simulink model "pmsg_wind_turbine_PI"  (R2022a)
settings: Solver=ode23tb  StartTime=0.0  StopTime=30  FixedStep=1e-4  MaxStep=1e-6  RelTol=1e-3
values from neighbouring files (symbols this model uses):
  Ci = 2878*10^-6    (= 0.002878)    [Completo.m]
  Lb = 0.9513*10^-3    (= 0.0009513)    [Completo.m]
  time = dados.Time;n    [Completo.m]
  vwind = dados.Vvento    [Completo.m]
undefined symbols (not defined in the file or in its folder): sigbuilder_block
libraries: spsCurrentMeasurementLib x3, eePowerMeasurement x3, spsVoltageMeasurementLib x3, spsSeriesRLCBranchLib x2, spsDCVoltageSourceLib x1, spsDiodeLib x1, spsMosfetLib x1, slpidlib x1, spsPWMGeneratorDCDCLib x1, spsPermanentMagnetSynchronousMachineLib x1, spsThreePhaseVIMeasurementLib x1, spsUniversalBridgeLib x1
settings Model: Creator=Taysa Banik  LastModifiedBy=LICON
settings SolverCC: ZeroCrossAlgorithm=Adaptive
settings DebuggingCC: MaxConsecutiveZCsMsg=warning  MaskedZcDiagnostic=none  IgnoredZcDiagnostic=none  MultiTaskCondExecSysMsg=warning  MultiTaskRateTransMsg=warning  ModelReferenceExtraNoncontSigs=warning

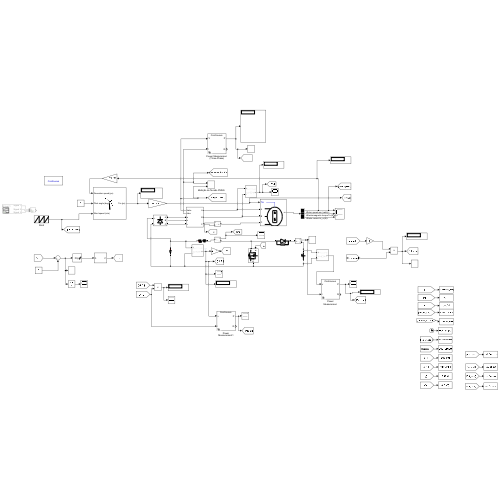
[thumbnail: Simulink's stored preview of the top-level diagram]
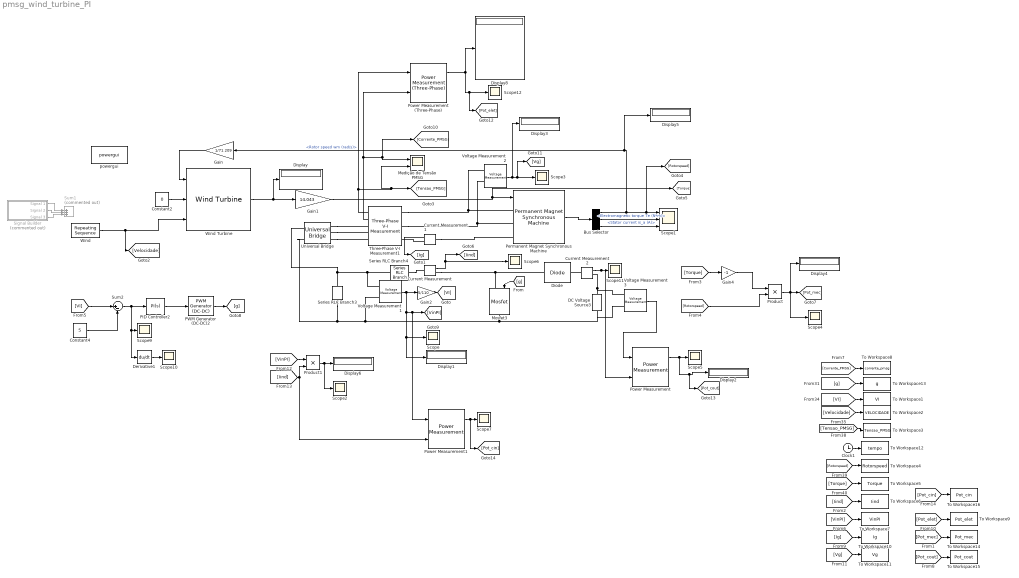
== system pmsg_wind_turbine_PI ==
  Bus Selector : BusSelector  OutputSignals=Rotor speed wm (rad/s),Electromagnetic torque Te (N*m),Stator current is_a (A)
  Clock1 : Clock
  Constant2 : Constant  Value=0
  Constant4 : Constant  Value=5
  Current Measurement : spsCurrentMeasurementLib/Current Measurement  PhasorSimulation=off  OutputType=Complex  PSBequivalent=0
  Current Measurement1 : spsCurrentMeasurementLib/Current Measurement  PhasorSimulation=off  OutputType=Complex  PSBequivalent=0
  Current Measurement2 : spsCurrentMeasurementLib/Current Measurement  PhasorSimulation=off  OutputType=Complex  PSBequivalent=0
  DC Voltage Source3 : spsDCVoltageSourceLib/DC Voltage Source  Amplitude=400  Measurements=Voltage
  Derivative1 : Derivative
  Diode : spsDiodeLib/Diode  Ron=0.001  Lon=0  Vf=0.1  IC=0  UseSnubber=0  Rs=50000  Cs=inf  Measurements=off
  Display{,1..6,8} (8 alike) : Display
  Gain : Gain  Gain=1/71.209
  Gain1 : Gain  Gain=14.043
  Gain2 : Gain  Gain=5/110
  Gain4 : Gain  Gain=-1
  Medição de Tensão PMSG : Scope  NumInputPorts=2
  Mosfet3 : spsMosfetLib/Mosfet  Ron=0.001  Lon=0  Rd=0.01  Vfd=0  IC=0  Rs=1e5  Cs=inf  Measurements=off
  PID Controller2 : slpidlib/PID Controller  Controller=PI  Form=Parallel  TimeDomain=Continuous-time  UseExternalTs=off  SampleTime=-1  IntegratorMethod=Forward Euler  FilterMethod=Forward Euler  ControllerParametersSource=internal  P=0.1928  I=11.6277  UseKiTs=off  D=0  N=100  UseFilter=on  TunerSelectOption=Frequency Response Based  InitialConditionSource=internal  InitialConditionForIntegrator=0  InitialConditionForFilter=0  DifferentiatorICPrevScaledInput=0  ExternalReset=none  TrackingMode=off  Kt=1  LimitOutput=on  SatLimitsSource=internal  UpperSaturationLimit=0.95  LowerSaturationLimit=0  LinearizeAsGain=on  AntiWindupMode=none  Kb=1  POutMin=[]  POutMax=[]  IOutMin=[]  IOutMax=[]  DOutMin=[]  DOutMax=[]  NOutMin=[]  NOutMax=[]  SumOutMin=[]  SumOutMax=[]  SaturationOutMin=[]  SaturationOutMax=[]  PParamMin=[]  PParamMax=[]  IParamMin=[]  IParamMax=[]  DParamMin=[]  DParamMax=[]  NParamMin=[]  NParamMax=[]  KbParamMin=[]  KbParamMax=[]  KtParamMin=[]  KtParamMax=[]  KbOutMin=[]  KbOutMax=[]  KtOutMin=[]  KtOutMax=[]  IntegratorOutMin=[]  IntegratorOutMax=[]  FilterOutMin=[]  FilterOutMax=[]  SumI1OutMin=[]  SumI1OutMax=[]  SumI2OutMin=[]  SumI2OutMax=[]  SumI3OutMin=[]  SumI3OutMax=[]  SumI4OutMin=[]  SumI4OutMax=[]  SumDOutMin=[]  SumDOutMax=[]  DifferentiatorOutMin=[]  DifferentiatorOutMax=[]  FilterDiffOutCoefMin=[]  FilterDiffOutCoefMax=[]  ReciprocalOutMin=[]  ReciprocalOutMax=[]  SumDenOutMin=[]  SumDenOutMax=[]  SumNumOutMin=[]  SumNumOutMax=[]  DivideOutMin=[]  DivideOutMax=[]  UdiffTsProdOutMin=[]  UdiffTsProdOutMax=[]  NTsProdOutMin=[]  NTsProdOutMax=[]  UintegralTsProdOutMin=[]  UintegralTsProdOutMax=[]  UngainTsProdOutMin=[]  UngainTsProdOutMax=[]  IntegratorContinuousStateAttributes=''  IntegratorStateMustResolveToSignalObject=off  IntegratorRTWStateStorageClass=Auto  FilterContinuousStateAttributes=''  FilterStateMustResolveToSignalObject=off  FilterRTWStateStorageClass=Auto  ParallelPVariant=InternalParameters  IdealPVariant=Disabled  IVariant=InternalParameters  DVariant=Disabled  IntegratorVariant=Continuous  SatVariant=Enabled  AWVariant=Passthrough  PCopyVariant=Disabled  TRVariant=Disabled  FdbkBlocksVariant=Forward  IdealPFdbkVariant=Disabled  SatFdbkVariant=Disabled  DerivativeFilterVariant=Disabled  NVariant=Disabled  NCopyVariant=Disabled_SignalSpec  FilterICVariant=Disabled  IntegratorICVariant=InternalICs  ExternalResetVariant=Disabled  TRSumVariant=Passthrough  SumFdbkVariant=Disabled  SumVariant=Sum_PI  TsampFilterVariant=InternalTs  TsampNgainVariant=Passthrough  TsampIntegralVariant=Passthrough  ExternalSaturationOutDataTypeStr=Inherit: Same as second input  aMode=0
  PWM Generator (DC-DC)2 : spsPWMGeneratorDCDCLib/PWM Generator (DC-DC)  Fsw=30000  Ts=1e-6
  Permanent Magnet Synchronous Machine : spsPermanentMagnetSynchronousMachineLib/Permanent Magnet Synchronous Machine  NbPhases=3  FluxDistribution=Sinusoidal  RotorType=Round  MechanicalLoad=Torque Tm  PresetModel=No  ShowDetailedParameters=on  MeasurementBus=off  Resistance=0.732  Inductance=8.5e-3  dqInductances=[8.5e-3,8.5e-3]  La=3.5e-3  MachineConstant=Voltage Constant (V_peak L-L / krpm)  Flux=0.13618  VoltageCst=172.9  TorqueCst=1.4299  Flat=120  Mechanical=[1E-3 1.79E-4 7 1E-3]  PolePairs=4  InitialConditions=[42.72,0, 0,0]  InitialConditions5ph=[0 0 0 0 0 0]  RefAngle=Aligned with phase A axis (original Park)  IterativeDiscreteModel=Trapezoidal non iterative  TsBlock=-1  TsPowergui=0
  Power Measurement : eePowerMeasurement/Power Measurement  LabelModeActiveChoice=Continuous  F=79.33  K=[0]  Ts=0
      settings: SourceProductBaseCode=PS
  Power Measurement1 : eePowerMeasurement/Power Measurement  LabelModeActiveChoice=Continuous  F=79.33  K=[0]  Ts=0
      settings: SourceProductBaseCode=PS
  Power Measurement (Three-Phase) : eePowerMeasurement/Power Measurement (Three-Phase)  LabelModeActiveChoice=Continuous  F=79.33  K=[0 1 2 3]  Seq=Positive  Ts=0
      settings: SourceProductBaseCode=PS
  Product : Product
  Product1 : Product
  Scope{,2..7,9..12} (11 alike) : Scope
  Scope1 : Scope  NumInputPorts=3
  Series RLC Branch3 : spsSeriesRLCBranchLib/Series RLC Branch  LConnTagsString=__new0  RConnTagsString=__new0  BranchType=C  Resistance=1  Inductance=1e-3  SetiL0=off  InitialCurrent=0  Capacitance=Ci  Setx0=on  InitialVoltage=100  Measurements=None
  Series RLC Branch4 : spsSeriesRLCBranchLib/Series RLC Branch  LConnTagsString=__new0  RConnTagsString=__new0  BranchType=RL  Resistance=1  Inductance=Lb  SetiL0=off  InitialCurrent=0  Capacitance=1e-3  Setx0=off  InitialVoltage=0  Measurements=None
  Signal Builder : Subsystem  Tag=STV Subsys  Commented=on  LoadFcn=sigbuilder_block('load');  StartFcn=sigbuilder_block('start');  StopFcn=sigbuilder_block('stop');  ClipboardFcn=sigbuilder_block('clipboard');  mask(Sigbuilder block){tuvar=[0:10]}
      mask help: Simulink:masks:SigbuilderBlock_MD
      mask init:
      | if ~strcmp(get_param(bdroot(gcbh),'SimulationStatus'),'stopped') tuvar = sigbuilder_block('maskInit'); end
      settings: CopyFcn=sigbuilder_block('copy');  DeleteFcn=sigbuilder_block('delete');  ModelCloseFcn=sigbuilder_block('modelClose');  PreSaveFcn=sigbuilder_block('preSave');  PauseFcn=sigbuilder_block('pause');  ContinueFcn=sigbuilder_block('continue');  NameChangeFcn=sigbuilder_block('namechange');  OpenFcn=sigbuilder_block('open',[61.5 90 1012.5 506.25 ]);  CloseFcn=sigbuilder_block('close');
      mask Display: plot(0, 0, 100, 100,[2, 2, 32, 32, 2], [68, 8, 8, 68, 68],[32, 2], [38, 38], [32, 19, 2],[53, 60, 44], [32, 17, 17, 2],[16, 16, 31, 31]);txt = getActiveGroup(gcbh);text(2, 100, txt,'verticalAlignment', 'top');
  Sum1 : Sum  Commented=on  Inputs=|+++
  Sum2 : Sum  Inputs=|+-
  Three-Phase V-I Measurement1 : spsThreePhaseVIMeasurementLib/Three-Phase V-I Measurement  VoltageMeasurement=phase-to-phase  SetLabelV=off  LabelV=Vabc  Vpu=off  VpuLL=off  CurrentMeasurement=yes  SetLabelI=off  LabelI=Iabc  Ipu=off  Pbase=100e6  Vbase=500e3  OutputType=Complex  PhasorSimulation=off  PSBequivalent=0
  To Workspace1 : ToWorkspace  VariableName=VI  SampleTime=1e-6
  To Workspace10 : ToWorkspace  VariableName=Ig  SampleTime=1e-6
  To Workspace11 : ToWorkspace  VariableName=Vg  SampleTime=1e-6
  To Workspace12 : ToWorkspace  VariableName=tempo  SampleTime=1e-6
  To Workspace13 : ToWorkspace  VariableName=g  SampleTime=1e-6
  To Workspace14 : ToWorkspace  VariableName=Pot_mec  SampleTime=1e-6
  To Workspace15 : ToWorkspace  VariableName=Pot_cout  SampleTime=1e-6
  To Workspace16 : ToWorkspace  VariableName=Pot_cin  SampleTime=1e-6
  To Workspace2 : ToWorkspace  VariableName=VELOCIDADE  SampleTime=1e-6
  To Workspace3 : ToWorkspace  VariableName=Tensao_PMSG  SampleTime=1e-6
  To Workspace4 : ToWorkspace  VariableName=Rotorspeed  SampleTime=1e-6
  To Workspace5 : ToWorkspace  VariableName=Torque  SampleTime=1e-6
  To Workspace6 : ToWorkspace  VariableName=Iind  SampleTime=1e-6
  To Workspace7 : ToWorkspace  VariableName=VinPI  SampleTime=1e-6
  To Workspace8 : ToWorkspace  VariableName=corrente_pmsg  SampleTime=1e-6
  To Workspace9 : ToWorkspace  VariableName=Pot_elet  SampleTime=1e-6
  Universal Bridge : spsUniversalBridgeLib/Universal Bridge  Arms=3  SnubberResistance=100000  SnubberCapacitance=inf  Device=Diodes  Ron=1e-3  Lon=0  ForwardVoltages="[  0  0  ]"  ForwardVoltage=0.1  GTOparameters=[ 10e-6 , 20e-6 ]  IGBTparameters=[ 1e-6 , 2e-6 ]  Measurements=None  Measurements_2=None  converterType=Rectifier
  Voltage Measurement1 : spsVoltageMeasurementLib/Voltage Measurement  PhasorSimulation=off  OutputType=Complex  PSBequivalent=0
  Voltage Measurement2 : spsVoltageMeasurementLib/Voltage Measurement  PhasorSimulation=off  OutputType=Complex  PSBequivalent=0
  Voltage Measurement3 : spsVoltageMeasurementLib/Voltage Measurement  PhasorSimulation=off  OutputType=Complex  PSBequivalent=0
  Wind : simulink/Sources/Repeating Sequence  rep_seq_t=[time]  rep_seq_y=[vwind]
  Wind Turbine : spsWindTurbineLib/Wind Turbine  Pnom=1000  Pelec_base=1000  wind_base=12  P_wind_base=1  speed_nom=1  pitch_angle=0  c1_c6="[0.51763          116          0.4            5           21     0.006795]"  cp_nom=0.48  lambda_nom=8.1
      settings: SourceProductBaseCode=PS
  powergui : spspowerguiLib/powergui  Priority=1  SimulationMode=Continuous  SampleTime=50e-6  frequency=60  Iterations=50  frequencyindice=0  Pbase=100e6  ErrMax=1e-4  UnitsV=kV  UnitsW=MW  buscounter=0  FunctionMessages=off  echomessages=off  EnableUseOfTLC=off  CurrentSourceSwitches=off  DisableSnubberDevices=off  DisableRonSwitches=off  DisableVfSwitches=off  DisplayEquations=off  AutomaticDiscreteSolvers=off  SolverType=Tustin/Backward Euler (TBE)  Interpol=off  ExternalGateDelay=off  methode=off  Ts=100  x0status=blocks  SPID=on  SwTol=0  HookPort=off  NonlinearTolerance=1e-4  nMaxIteration=100  ContinueOnMaxIteration=off  RestoreLinks=warning  ResistiveCurrentMeasurement=off  Frange=[0:2:500]  Ylog=off  Xlog=on  ShowGrid=off  save=off  variable=ZData  structure=0  ZoomFFT=off  StartTime=0.0  cycles=1  DisplayStyle=1  fundamental=60  FreqAxis=off  MaxFrequency=1000  frequencyindicesteady=1  RmsSteady=1  display=off
  wires:
  Constant2/1 -> Wind Turbine/2
  Three-Phase V-I Measurement1/1 -> Power Measurement (Three-Phase)/1, Medição de Tensão PMSG/2, [Tensao_PMSG]
  Permanent Magnet Synchronous Machine/1 -> Bus Selector/1
  Bus Selector/1 -> [Rotorspeed], Scope1/1, Display5/1, Gain/1  "<Rotor speed wm (rad/s)>"
  Bus Selector/2 -> Scope1/2  "<Electromagnetic torque Te (N*m)>"
  Bus Selector/3 -> Scope1/3  "<Stator current is_a (A)>"
  Gain/1 -> Wind Turbine/1
  Wind Turbine/1 -> Display/1, Gain1/1
  Gain1/1 -> Permanent Magnet Synchronous Machine/1, [Torque]
  Voltage Measurement1/1 -> Gain2/1, Power Measurement1/1, [VinPI], Scope/1, Display1/1
  [g] -> Mosfet3/1
  Gain2/1 -> [VI]
  Signal Builder/1(Signal 1) -> Sum1/1
  Signal Builder/2(Signal 2) -> Sum1/2
  Signal Builder/3(Signal 3) -> Sum1/3
  [VI] -> To Workspace1/1
  [g] -> To Workspace13/1
  [Torque] -> To Workspace5/1
  [Velocidade] -> To Workspace2/1
  Clock1/1 -> To Workspace12/1
  [Tensao_PMSG] -> To Workspace3/1
  [Rotorspeed] -> To Workspace4/1
  Current Measurement/1 -> [Iind], Scope6/1
  [Iind] -> To Workspace6/1
  Product/1 -> Display4/1, Scope4/1, [Pot_mec]
  [Rotorspeed] -> Product/2
  [Torque] -> Gain4/1
  Gain4/1 -> Product/1
  Constant4/1 -> Sum2/2
  [VI] -> Sum2/1
  PID Controller2/1 -> PWM Generator (DC-DC)2/1
  Derivative1/1 -> Scope10/1
  PWM Generator (DC-DC)2/1 -> [g]
  Sum2/1 -> Derivative1/1, Scope9/1, PID Controller2/1
  [VinPI] -> To Workspace7/1
  [Corrente_PMSG] -> To Workspace8/1
  [Pot_elet] -> To Workspace9/1
  Current Measurement1/1 -> [Ig]
  Voltage Measurement2/1 -> Display3/1, [Vg], Scope3/1
  [Vg] -> To Workspace11/1
  [Ig] -> To Workspace10/1
  [Pot_mec] -> To Workspace14/1
  Current Measurement2/1 -> Power Measurement/2, Scope11/1
  Power Measurement (Three-Phase)/1 -> [Pot_elet], Scope12/1, Display8/1
  Three-Phase V-I Measurement1/2 -> Power Measurement (Three-Phase)/2, Medição de Tensão PMSG/1, [Corrente_PMSG]
  Voltage Measurement3/1 -> Power Measurement/1
  Power Measurement/1 -> [Pot_cout], Display2/1, Scope5/1
  [Pot_cout] -> To Workspace15/1
  [Iind] -> Product1/2, Power Measurement1/2
  Product1/1 -> Scope2/1, Display6/1
  Wind/1 -> [Velocidade], Wind Turbine/3
  [VinPI] -> Product1/1
  Power Measurement1/1 -> [Pot_cin], Scope7/1
  [Pot_cin] -> To Workspace16/1
  connections:
  Three-Phase V-I Measurement1/LConn1 -- Voltage Measurement2/LConn1 -- Permanent Magnet Synchronous Machine/LConn1
  Three-Phase V-I Measurement1/LConn2 -- Voltage Measurement2/LConn2 -- Permanent Magnet Synchronous Machine/LConn2
  Universal Bridge/LConn1 -- Three-Phase V-I Measurement1/RConn1
  Universal Bridge/LConn2 -- Three-Phase V-I Measurement1/RConn2
  Universal Bridge/LConn3 -- Three-Phase V-I Measurement1/RConn3
  Mosfet3/LConn1 -- Current Measurement/RConn1 -- Diode/LConn1
  Voltage Measurement1/LConn1 -- Series RLC Branch4/LConn1 -- Universal Bridge/RConn1 -- Series RLC Branch3/LConn1
  Series RLC Branch3/RConn1 -- Universal Bridge/RConn2 -- Voltage Measurement1/LConn2 -- Voltage Measurement3/LConn2 -- DC Voltage Source3/LConn1 -- Mosfet3/RConn1
  Current Measurement1/LConn1 -- Permanent Magnet Synchronous Machine/LConn3
  Current Measurement1/RConn1 -- Three-Phase V-I Measurement1/LConn3
  Series RLC Branch4/RConn1 -- Current Measurement/LConn1
  Current Measurement2/LConn1 -- Diode/RConn1
  DC Voltage Source3/RConn1 -- Current Measurement2/RConn1 -- Voltage Measurement3/LConn1

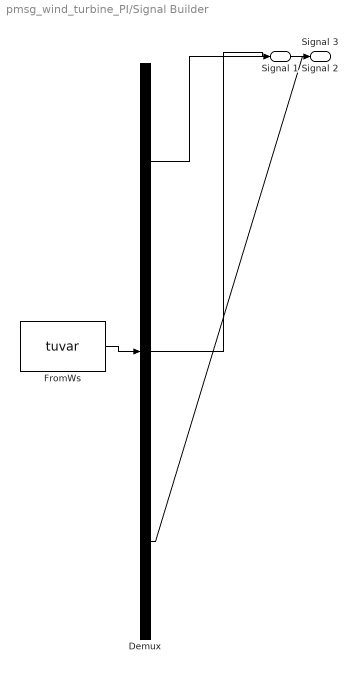
== system pmsg_wind_turbine_PI/Signal Builder ==
  Demux : Demux  Tag=STV Demux  Outputs=3
      settings: DisplayOption=none
  FromWs : FromWorkspace  Tag=STV FromWs  VariableName=tuvar
      SigBuilderData=|
      | common.afterFinalStr = 'Extrapolate'
      | common.sampleTime = 0
      | dataSet.timeRange = [0 10]
      | dataSet.name = 'Group 1'
      | sbobj.Groups.Name = 'Group 1'
      | sbobj.Groups.Signals(1).Name = 'Signal 1'
      | sbobj.Groups.Signals(1).XData = [0 1.5 1.5 6 10]
      | sbobj.Groups.Signals(1).YData = [12 12 0 0 0]
      | sbobj.Groups.Signals(2).Name = 'Signal 2'
      | sbobj.Groups.Signals(2).XData = [0 1.5 1.5 2.5 2.5 10]
      | sbobj.Groups.Signals(2).YData = [0 0 10 10 0 0]
      | sbobj.Groups.Signals(3).Name = 'Signal 3'
      | sbobj.Groups.Signals(3).XData = [0 2.5 2.5 10]
      | sbobj.Groups.Signals(3).YData = [0 0 12 12]
  Signal 1 : Outport  Tag=STV Outport
  Signal 2 : Outport  Tag=STV Outport  Port=2
  Signal 3 : Outport  Tag=STV Outport  Port=3
  wires:
  Demux/1 -> Signal 1/1
  FromWs/1 -> Demux/1
  Demux/2 -> Signal 2/1
  Demux/3 -> Signal 3/1
